simulink model "Part_Extra_Question"  (R2016a)
settings: Solver=VariableStepAuto  StartTime=0.0  StopTime=20  RelTol=1e-3
values from neighbouring files (symbols this model uses):
  Alpha = 1    [Parameters_And_Plot.m]    (also in Part5_Specified_Destinations.m)
  K12 = K(1,2)    [Parameters_And_Plot.m]    (also in Part5_Specified_Destinations.m)
  K13 = K(1,3)    [Parameters_And_Plot.m]    (also in Part5_Specified_Destinations.m)
  K14 = K(1,4)    [Parameters_And_Plot.m]    (also in Part5_Specified_Destinations.m)
  K15 = K(1,5)    [Parameters_And_Plot.m]    (also in Part5_Specified_Destinations.m)
  K21 = K(2,1)    [Parameters_And_Plot.m]    (also in Part5_Specified_Destinations.m)
  K23 = K(2,1)    [Parameters_And_Plot.m]    (also in Part5_Specified_Destinations.m)
  K24 = K(2,1)    [Parameters_And_Plot.m]    (also in Part5_Specified_Destinations.m)
  K25 = K(2,1)    [Parameters_And_Plot.m]    (also in Part5_Specified_Destinations.m)
  K31 = K(3,1)    [Parameters_And_Plot.m]    (also in Part5_Specified_Destinations.m)
  K32 = K(3,2)    [Parameters_And_Plot.m]    (also in Part5_Specified_Destinations.m)
  K34 = K(3,4)    [Parameters_And_Plot.m]    (also in Part5_Specified_Destinations.m)
  K35 = K(3,5)    [Parameters_And_Plot.m]    (also in Part5_Specified_Destinations.m)
  K41 = K(4,1)    [Parameters_And_Plot.m]    (also in Part5_Specified_Destinations.m)
  K42 = K(4,2)    [Parameters_And_Plot.m]    (also in Part5_Specified_Destinations.m)
  K43 = K(4,3)    [Parameters_And_Plot.m]    (also in Part5_Specified_Destinations.m)
  K45 = K(4,5)    [Parameters_And_Plot.m]    (also in Part5_Specified_Destinations.m)
  K51 = K(5,1)    [Parameters_And_Plot.m]    (also in Part5_Specified_Destinations.m)
  K52 = K(5,2)    [Parameters_And_Plot.m]    (also in Part5_Specified_Destinations.m)
  K53 = K(5,3)    [Parameters_And_Plot.m]    (also in Part5_Specified_Destinations.m)
  K54 = K(5,4)    [Parameters_And_Plot.m]    (also in Part5_Specified_Destinations.m)
  L = 1    [Parameters_And_Plot.m]    (also in Part5_Specified_Destinations.m)
  x1_0 = r1_0(1)    [Parameters_And_Plot.m]    (also in Part5_Specified_Destinations.m)
  x1d = r1d(1)    [Parameters_And_Plot.m]    (also in Part5_Specified_Destinations.m)
  x2_0 = r2_0(1)    [Parameters_And_Plot.m]    (also in Part5_Specified_Destinations.m)
  x2d = r2d(1)    [Parameters_And_Plot.m]    (also in Part5_Specified_Destinations.m)
  x3_0 = r3_0(1)    [Parameters_And_Plot.m]    (also in Part5_Specified_Destinations.m)
  x3d = r3d(1)    [Parameters_And_Plot.m]    (also in Part5_Specified_Destinations.m)
  x4_0 = r4_0(1)    [Parameters_And_Plot.m]    (also in Part5_Specified_Destinations.m)
  x4d = r4d(1)    [Parameters_And_Plot.m]    (also in Part5_Specified_Destinations.m)
  x5_0 = r5_0(1)    [Parameters_And_Plot.m]    (also in Part5_Specified_Destinations.m)
  x5d = r5d(1)    [Parameters_And_Plot.m]    (also in Part5_Specified_Destinations.m)
  y1_0 = r1_0(2)    [Parameters_And_Plot.m]    (also in Part5_Specified_Destinations.m)
  y1d = r1d(2)    [Parameters_And_Plot.m]    (also in Part5_Specified_Destinations.m)
  y2_0 = r2_0(2)    [Parameters_And_Plot.m]    (also in Part5_Specified_Destinations.m)
  y2d = r2d(2)    [Parameters_And_Plot.m]    (also in Part5_Specified_Destinations.m)
  y3_0 = r3_0(2)    [Parameters_And_Plot.m]    (also in Part5_Specified_Destinations.m)
  y3d = r3d(2)    [Parameters_And_Plot.m]    (also in Part5_Specified_Destinations.m)
  y4_0 = r4_0(2)    [Parameters_And_Plot.m]    (also in Part5_Specified_Destinations.m)
  y4d = r4d(2)    [Parameters_And_Plot.m]    (also in Part5_Specified_Destinations.m)
  y5_0 = r5_0(2)    [Parameters_And_Plot.m]    (also in Part5_Specified_Destinations.m)
  y5d = r5d(2)    [Parameters_And_Plot.m]    (also in Part5_Specified_Destinations.m)
settings Model: Creator=Mohammad Hammoud  LastModifiedBy=Mohammad Hammoud

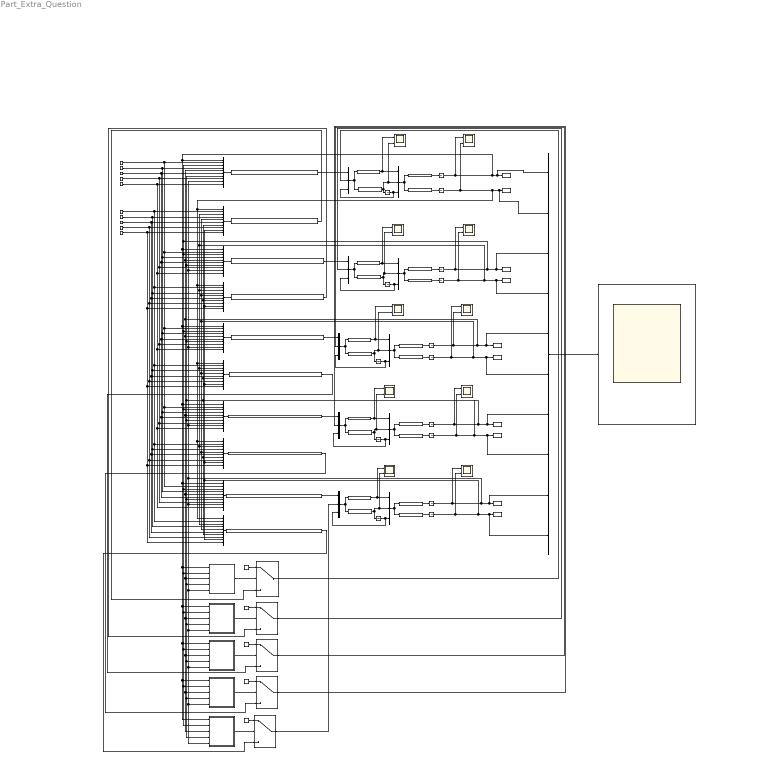
== system Part_Extra_Question ==
  note: C
  note: Test-Robot 1
  note: < Robot 1
  note: In this Model, after the 5 Robots reach their Final Destination, they change direction, and
      | continue their trajectory parallel to the y-axis with a constant inter-distance between them
  note: Yi desired
  note: Xi desired
  note: These Matlab Functions (IF conditions on x positions) test if all robots arrive to their final destinations;
      | If this condition is validated, then all Uyi become Constant = 2 (in our case, can be changed if we wand to change the speed of the robots in this new trajectory - parallel to the y-axis),
      | If not, the control law Uyi maintains the same to the moment of reaching each robot his final destination.
      |
      | This operation of switching the Uyi value between the constant 2 or to be maintained is accomplished by using SWITCHES with the condition confirmed in the Previous Matlab Function.
  note: Consensus-based Conrol Law
  note: Scope to show all Linear Displacements Xi and Yi of All Robots, function of Time
  note: In these Scopes we can see the Graphs of Linear Velocity Vi and Angular Velocity Wi for each Robot alone
  note: Extra Question: " Propose a controller that forms the platoon, then the robots continue to travel in platooning, parallel to the
      | 'y-axis' at constant speed. So the platoon change direction, but the inter-distance between robots should be maintained "
  note: R q : We want to change the direction of the robots after arriving to their desired destination, by continue moving parallel to the y-axis .
      | At a certain time ta, Xi and Yi will converge to their correspondant desired values Xid and Yid respectively. For t > ta, Xi is constant and Yi is increased linearly by switching Uyi to a constant value and thus Yi = C.t. Therefore, the robot will continue to move vertically.
      | As C increases, the speed of moving parallel to y axis increases.
  note: Uy3
  note: Uy4
  note: Uy5
  note: Uy2
  note: x1
  note: In these Scopes we can see the Graphs of Linear displacements Xi and Yi for each Robot alone
  note: < Robot 2
  note: < Robot 3
  note: < Robot 4
  note: < Robot 5
  note: Test-Robot 2
  note: Test-Robot 3
  note: Test-Robot 4
  note: Test-Robot 5
  Constant{,1..2,13..14} (5 alike) : Constant  Value=2
  Constant10 : Constant  Value=y3d
  Constant11 : Constant  Value=y4d
  Constant12 : Constant  Value=y5d
  Constant3 : Constant  Value=x1d
  Constant4 : Constant  Value=x2d
  Constant5 : Constant  Value=x3d
  Constant6 : Constant  Value=x4d
  Constant7 : Constant  Value=x5d
  Constant8 : Constant  Value=y1d
  Constant9 : Constant  Value=y2d
  Integrator{,1,4,6,10} (5 alike) : Integrator
  "Integrator1 " : Integrator  InitialCondition=x1_0
  "Integrator10 " : Integrator  InitialCondition=y4_0
  "Integrator11 " : Integrator  InitialCondition=x5_0
  "Integrator12 " : Integrator  InitialCondition=y5_0
  Integrator2 : Integrator  InitialCondition=y1_0
  Integrator3 : Integrator  InitialCondition=y2_0
  "Integrator4 " : Integrator  InitialCondition=x2_0
  "Integrator5 " : Integrator  InitialCondition=x3_0
  "Integrator8 " : Integrator  InitialCondition=y3_0
  "Integrator9 " : Integrator  InitialCondition=x4_0
  MATLAB Function : MATLAB Function  TreatAsAtomicUnit=on
  MATLAB Function1 : MATLAB Function  TreatAsAtomicUnit=on
  MATLAB Function2 : MATLAB Function  TreatAsAtomicUnit=on
  MATLAB Function3 : MATLAB Function  TreatAsAtomicUnit=on
  MATLAB Function4 : MATLAB Function  TreatAsAtomicUnit=on
  Mux{,1..4,7,10,13,16..17,20} (11 alike) : Mux  Inputs=10
  Mux{5..6,8..9,11..12,14..15,21..22} (10 alike) : Mux  Inputs=3
  Scope : Scope
  Scope{1..10} (10 alike) : Scope  NumInputPorts=2
  Switch{,1..4} (5 alike) : Switch  Criteria=u2 > Threshold  Threshold=5
  To Workspace1 : ToWorkspace  VariableName=xh1  SampleTime=-1
  To Workspace11 : ToWorkspace  VariableName=xh3  SampleTime=-1
  To Workspace12 : ToWorkspace  VariableName=yh3  SampleTime=-1
  To Workspace2 : ToWorkspace  VariableName=yh1  SampleTime=-1
  To Workspace3 : ToWorkspace  VariableName=xh2  SampleTime=-1
  To Workspace4 : ToWorkspace  VariableName=yh2  SampleTime=-1
  To Workspace5 : ToWorkspace  VariableName=xh5  SampleTime=-1
  To Workspace6 : ToWorkspace  VariableName=xh4  SampleTime=-1
  To Workspace7 : ToWorkspace  VariableName=yh4  SampleTime=-1
  To Workspace8 : ToWorkspace  VariableName=yh5  SampleTime=-1
  Ux1 : Fcn  Expr=-Alpha*(u(1)-u(2))-K12*((u(1)-u(2))-(u(3)-u(4)))-K13 * ((u(1) - u(2)) - (u(5) - u(6))) - K14 * ((u(1) - u(2)) - (u(7) - u(8))) - K15 * ((u(1) - u(2)) - (u(9) - u(10)))
  Ux2 : Fcn  Expr=-Alpha * (u(3) - u(4)) - K21 * ((u(3) - u(4)) - (u(1) - u(2))) - K23 * ((u(3) - u(4)) - (u(5) - u(6))) - K24 * ((u(3) - u(4)) - (u(7) - u(8))) - K25 * ((u(3) - u(4)) - (u(9) - u(10)))
  Ux3 : Fcn  Expr=-Alpha * (u(5) - u(6)) - K31 * ((u(5) - u(6)) - (u(1) - u(2))) - K32 * ((u(5) - u(6)) - (u(3) - u(4))) - K34 * ((u(5) - u(6)) - (u(7) - u(8))) - K35 * ((u(5) - u(6)) - (u(9) - u(10)))
  Ux4 : Fcn  Expr=-Alpha * (u(7) - u(8)) - K41 * ((u(7) - u(8)) - (u(1) - u(2))) - K42 * ((u(7) - u(8)) - (u(3) - u(4))) - K43 * ((u(7) - u(8)) - (u(5) - u(6))) - K45 * ((u(7) - u(8)) - (u(9) - u(10)))
  Ux5 : Fcn  Expr=-Alpha * (u(9) - u(10)) - K51 * ((u(9) - u(10)) - (u(1) - u(2))) - K52 * ((u(9) - u(10)) - (u(3) - u(4))) - K53 * ((u(9) - u(10)) - (u(5) - u(6))) - K54 * ((u(9) - u(10)) - (u(7) - u(8)))
  Uy1 : Fcn  Expr=-Alpha*(u(1)-u(2))-K12*((u(1)-u(2))-(u(3)-u(4)))-K13 * ((u(1) - u(2)) - (u(5) - u(6))) - K14 * ((u(1) - u(2)) - (u(7) - u(8))) - K15 * ((u(1) - u(2)) - (u(9) - u(10)))
  Uy2 : Fcn  Expr=-Alpha * (u(3) - u(4)) - K21 * ((u(3) - u(4)) - (u(1) - u(2))) - K23 * ((u(3) - u(4)) - (u(5) - u(6))) - K24 * ((u(3) - u(4)) - (u(7) - u(8))) - K25 * ((u(3) - u(4)) - (u(9) - u(10)))
  Uy3 : Fcn  Expr=-Alpha * (u(5) - u(6)) - K31 * ((u(5) - u(6)) - (u(1) - u(2))) - K32 * ((u(5) - u(6)) - (u(3) - u(4))) - K34 * ((u(5) - u(6)) - (u(7) - u(8))) - K35 * ((u(5) - u(6)) - (u(9) - u(10)))
  Uy4 : Fcn  Expr=-Alpha * (u(7) - u(8)) - K41 * ((u(7) - u(8)) - (u(1) - u(2))) - K42 * ((u(7) - u(8)) - (u(3) - u(4))) - K43 * ((u(7) - u(8)) - (u(5) - u(6))) - K45 * ((u(7) - u(8)) - (u(9) - u(10)))
  Uy5 : Fcn  Expr=-Alpha * (u(9) - u(10)) - K51 * ((u(9) - u(10)) - (u(1) - u(2))) - K52 * ((u(9) - u(10)) - (u(3) - u(4))) - K53 * ((u(9) - u(10)) - (u(5) - u(6))) - K54 * ((u(9) - u(10)) - (u(7) - u(8)))
  V{1..5} (5 alike) : Fcn  Expr=u(1)*cos(u(3)) + u(2)*sin(u(3))
  W{1..5} (5 alike) : Fcn  Expr=-(u(1)*sin(u(3)))/L + (u(2)*cos(u(3)))/L
  Xhdot {1..5} (5 alike) : Fcn  Expr=u(1)*cos(u(3)) - L*u(2)*sin(u(3))
  Yhdot {1..5} (5 alike) : Fcn  Expr=u(1)*sin(u(3)) + L*u(2)*cos(u(3))
  wires:
  Constant3/1 -> Mux/2, Mux20/2, Mux10/2, Mux4/2, Mux3/2  "x1d"
  Mux/1 -> Ux1/1
  Constant4/1 -> Mux/4, Mux4/4, Mux3/4, Mux10/4, Mux20/4  "x2d"
  Constant5/1 -> Mux/6, Mux4/6, Mux3/6, Mux10/6, Mux20/6  "x3d"
  Constant6/1 -> Mux4/8, Mux3/8, Mux10/8, Mux20/8, Mux/8  "x4d"
  Constant7/1 -> Mux20/10, Mux4/10, Mux3/10, Mux10/10, Mux/10  "x5d"
  Constant8/1 -> Mux16/2, Mux13/2, Mux2/2, Mux7/2, Mux1/2  "y1d"
  Mux1/1 -> Uy1/1
  Constant9/1 -> Mux16/4, Mux13/4, Mux2/4, Mux7/4, Mux1/4  "y2d"
  Constant10/1 -> Mux16/6, Mux13/6, Mux2/6, Mux7/6, Mux1/6  "y3d"
  Constant11/1 -> Mux2/8, Mux16/8, Mux13/8, Mux7/8, Mux1/8  "y4d"
  Constant12/1 -> Mux16/10, Mux13/10, Mux2/10, Mux7/10, Mux1/10  "y5d"
  Mux2/1 -> Uy3/1
  Mux4/1 -> Ux5/1
  Mux5/1 -> V1/1, W1/1
  Integrator/1 -> Mux6/3, Mux5/3  "Theta 1"
  V1/1 -> Scope1/1, Mux6/1  "V1"
  W1/1 -> Scope1/2, Mux6/2, Integrator/1  "W1"
  Mux6/1 -> Xhdot 1/1, Yhdot 1/1
  Yhdot 1/1 -> Integrator2/1
  Xhdot 1/1 -> "Integrator1 "/1
  "Integrator1 "/1 -> Scope4/1, Mux/1, Mux3/1, MATLAB Function4/1(x1), MATLAB Function3/1(x1), MATLAB Function2/1(x1), MATLAB Function1/1(x1), MATLAB Function/1(x1), Mux4/1, Mux10/1, Mux20/1, Mux17/1, To Workspace1/1  "x1"
  Integrator2/1 -> Scope4/2, Mux1/1, Mux13/1, Mux16/1, Mux2/1, Mux7/1, Mux17/2, To Workspace2/1  "y1"
  Mux8/1 -> V2/1, W2/1
  Integrator1/1 -> Mux8/3, Mux9/3  "Theta 2"
  V2/1 -> Scope2/1, Mux9/1  "V2"
  W2/1 -> Integrator1/1, Scope2/2, Mux9/2  "W2"
  Mux9/1 -> Yhdot 2/1, Xhdot 2/1
  Yhdot 2/1 -> Integrator3/1
  Xhdot 2/1 -> "Integrator4 "/1
  "Integrator4 "/1 -> Scope3/1, Mux17/3, To Workspace3/1, MATLAB Function3/2(x2), MATLAB Function4/2(x2), MATLAB Function2/2(x2), MATLAB Function1/2(x2), MATLAB Function/2(x2), Mux4/3, Mux3/3, Mux10/3, Mux20/3, Mux/3  "x2"
  Integrator3/1 -> Scope3/2, Mux17/4, To Workspace4/1, Mux1/3, Mux7/3, Mux16/3, Mux13/3, Mux2/3  "y2"
  Uy3/1 -> Switch1/3  "Uy3"
  Mux20/1 -> Ux2/1
  Ux2/1 -> Mux8/1  "Ux2"
  Mux7/1 -> Uy2/1
  Mux10/1 -> Ux3/1
  Mux21/1 -> V3/1, W3/1
  Integrator10/1 -> Mux21/3, Mux22/3  "Theta 3"
  V3/1 -> Scope5/1, Mux22/1  "V3"
  W3/1 -> Integrator10/1, Scope5/2, Mux22/2  "W3"
  Mux22/1 -> Yhdot 3/1, Xhdot 3/1
  Yhdot 3/1 -> "Integrator8 "/1
  Xhdot 3/1 -> "Integrator5 "/1
  "Integrator5 "/1 -> MATLAB Function4/3(x3), MATLAB Function3/3(x3), MATLAB Function2/3(x3), MATLAB Function1/3(x3), MATLAB Function/3(x3), Mux4/5, Mux3/5, Mux10/5, Mux/5, Mux20/5, Mux17/5, To Workspace11/1, Scope6/2  "x3"
  "Integrator8 "/1 -> Scope6/1, Mux17/6, To Workspace12/1, Mux7/5, Mux1/5, Mux16/5, Mux13/5, Mux2/5  "y3"
  Ux3/1 -> Mux21/1  "Ux3"
  Mux3/1 -> Ux4/1
  Mux11/1 -> V4/1, W4/1
  Integrator4/1 -> Mux11/3, Mux12/3  "Theta 4"
  V4/1 -> Scope7/1, Mux12/1  "V4"
  W4/1 -> Integrator4/1, Mux12/2, Scope7/2  "W4"
  Mux12/1 -> Yhdot 4/1, Xhdot 4/1
  Yhdot 4/1 -> "Integrator10 "/1
  Xhdot 4/1 -> "Integrator9 "/1
  "Integrator9 "/1 -> Scope8/1, MATLAB Function4/4(x4), MATLAB Function3/4(x4), MATLAB Function2/4(x4), MATLAB Function1/4(x4), MATLAB Function/4(x4), Mux4/7, Mux3/7, Mux/7, Mux20/7, Mux10/7, Mux17/7, To Workspace6/1  "x4"
  "Integrator10 "/1 -> Scope8/2, Mux7/7, Mux1/7, Mux2/7, Mux16/7, Mux13/7, Mux17/8, To Workspace7/1  "y4"
  Ux4/1 -> Mux11/1  "Ux4"
  Mux13/1 -> Uy4/1
  Uy4/1 -> Switch3/3  "Uy4"
  Mux14/1 -> V5/1, W5/1
  Integrator6/1 -> Mux14/3, Mux15/3  "Theta 5"
  V5/1 -> Scope9/1, Mux15/1  "V5"
  W5/1 -> Integrator6/1, Mux15/2, Scope9/2  "W5"
  Mux15/1 -> Yhdot 5/1, Xhdot 5/1
  Yhdot 5/1 -> "Integrator12 "/1
  Xhdot 5/1 -> "Integrator11 "/1
  "Integrator11 "/1 -> Scope10/1, Mux/9, Mux20/9, Mux10/9, Mux3/9, MATLAB Function4/5(x5), MATLAB Function3/5(x5), MATLAB Function2/5(x5), MATLAB Function1/5(x5), MATLAB Function/5(x5), Mux4/9, Mux17/9, To Workspace5/1  "x5"
  "Integrator12 "/1 -> Mux1/9, Mux7/9, Mux2/9, Mux13/9, Mux16/9, Mux17/10, To Workspace8/1, Scope10/2  "y5"
  Ux5/1 -> Mux14/1  "Ux5"
  Mux16/1 -> Uy5/1
  Uy5/1 -> Switch4/3  "Uy5"
  Mux17/1 -> Scope/1
  MATLAB Function/1(Test_Arriving_First_Desired_Positions) -> Switch/2
  Constant/1 -> Switch/1
  Ux1/1 -> Mux5/1  "Ux1"
  Switch/1 -> Mux5/2  "Uy1"
  Uy1/1 -> Switch/3  "Uy1"
  MATLAB Function1/1(Test_Arriving_First_Desired_Positions) -> Switch2/2
  Constant1/1 -> Switch2/1
  Uy2/1 -> Switch2/3  "Uy2"
  Switch2/1 -> Mux8/2  "Uy2"
  MATLAB Function2/1(Test_Arriving_First_Desired_Positions) -> Switch1/2
  Constant2/1 -> Switch1/1
  Switch1/1 -> Mux21/2  "Uy3"
  MATLAB Function3/1(Test_Arriving_First_Desired_Positions) -> Switch3/2
  Constant13/1 -> Switch3/1
  Switch3/1 -> Mux11/2  "Uy4"
  MATLAB Function4/1(Test_Arriving_First_Desired_Positions) -> Switch4/2
  Constant14/1 -> Switch4/1
  Switch4/1 -> Mux14/2  "Uy5"

== matlab function Part_Extra_Question/MATLAB Function1 ==
  data: x1 input; Test_Arriving_First_Desired_Positions output; x2 input; x3 input; x4 input; x5 input
function Test_Arriving_First_Desired_Positions = fcn(x1,x2,x3,x4,x5)
%#codegen
if(x1>34.99999 && x2>31.99999 && x3>28.99999 && x4>25.99999 && x5>22.99999)
    Test_Arriving_First_Desired_Positions = 10;
else
    Test_Arriving_First_Desired_Positions = 0;
end

== matlab function Part_Extra_Question/MATLAB Function ==
  data: x1 input; Test_Arriving_First_Desired_Positions output; x2 input; x3 input; x4 input; x5 input
function Test_Arriving_First_Desired_Positions = fcn(x1,x2,x3,x4,x5)
%#codegen
if(x1>34.99999 && x2>31.99999 && x3>28.99999 && x4>25.99999 && x5>22.99999)
    Test_Arriving_First_Desired_Positions = 10;
else
    Test_Arriving_First_Desired_Positions = 0;
end

== matlab function Part_Extra_Question/MATLAB Function2 ==
  data: x1 input; Test_Arriving_First_Desired_Positions output; x2 input; x3 input; x4 input; x5 input
function Test_Arriving_First_Desired_Positions = fcn(x1,x2,x3,x4,x5)
%#codegen
if(x1>34.99999 && x2>31.99999 && x3>28.99999 && x4>25.99999 && x5>22.99999)
    Test_Arriving_First_Desired_Positions = 10;
else
    Test_Arriving_First_Desired_Positions = 0;
end

== matlab function Part_Extra_Question/MATLAB Function3 ==
  data: x1 input; Test_Arriving_First_Desired_Positions output; x2 input; x3 input; x4 input; x5 input
function Test_Arriving_First_Desired_Positions = fcn(x1,x2,x3,x4,x5)
%#codegen
if(x1>34.99999 && x2>31.99999 && x3>28.99999 && x4>25.99999 && x5>22.99999)
    Test_Arriving_First_Desired_Positions = 10;
else
    Test_Arriving_First_Desired_Positions = 0;
end

== matlab function Part_Extra_Question/MATLAB Function4 ==
  data: x1 input; Test_Arriving_First_Desired_Positions output; x2 input; x3 input; x4 input; x5 input
function Test_Arriving_First_Desired_Positions = fcn(x1,x2,x3,x4,x5)
%#codegen
if(x1>34.99999 && x2>31.99999 && x3>28.99999 && x4>25.99999 && x5>22.99999)
    Test_Arriving_First_Desired_Positions = 10;
else
    Test_Arriving_First_Desired_Positions = 0;
end
